simulink model "test3"  (Simulink 7.5)
settings: Solver=ode45  StartTime=0.0  StopTime=10.0  RelTol=1e-3
InitFcn:
  | %% DSPBuilder Start
  | alt_dspbuilder_update_model(bdroot)
  | %% DSPBuilder End
libraries: allblocks_alteradspbuilder2 x16
settings Model: Creator=Administrator  LastModifiedBy=Administrator

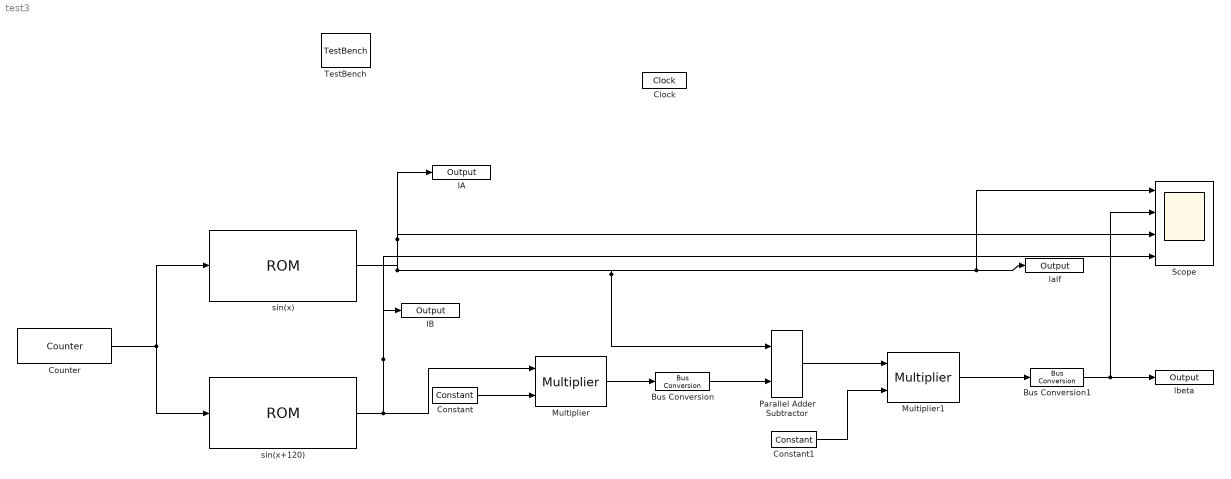
== system test3 ==
  Bus Conversion : allblocks_alteradspbuilder2/Bus Conversion  BusType=Signed Fractional  ibwl=18  ibwr=14  bwl=2  bwr=14  bitToConnectToOutputLSB=3  round=off  saturate=off  pipeline_display=0
  Bus Conversion1 : allblocks_alteradspbuilder2/Bus Conversion  BusType=Signed Fractional  ibwl=4  ibwr=28  bwl=2  bwr=14  bitToConnectToOutputLSB=3  round=off  saturate=off  pipeline_display=0
  Clock : allblocks_alteradspbuilder2/Clock  ClockPeriod=1/10000  ClockPeriodUnit=sec  SampleTime=1/10000  ResetLatency=0  ResetRegisterCascadeDepth=0  SimulationStartCycle=5  PhaseOffset=0  Reset=aclr  ResetType=Active Low  Export=off
  Constant : allblocks_alteradspbuilder2/Constant  mask_cst=2  BusType=Signed Integer  bwl=16  bwr=0  roundMode=Truncate  satMode=Wrap  SpecifyClock=off  allowFloatingPointOverride=on  logOutputs=off  logFile=C:\altera\13.1\quartus\dsp_builder\tb_test3\test3_Constant.fixedpointlog
  Constant1 : allblocks_alteradspbuilder2/Constant  mask_cst=sqrt(1/3)  BusType=Signed Fractional  bwl=2  bwr=14  roundMode=Truncate  satMode=Wrap  SpecifyClock=off  allowFloatingPointOverride=on  logOutputs=off  logFile=C:\altera\13.1\quartus\dsp_builder\tb_test3\test3_Constant1.fixedpointlog
  Counter : allblocks_alteradspbuilder2/Counter  BusType=Unsigned Integer  bwl=12  bwr=0  use_modulo=on  modulo=4096  SpecifyClock=off  direction=Increment  use_sload=off  use_sset=off  svalue=1  use_clk_ena=off  use_ena=off  use_sclr=off  pipeline_display=1
  IA : allblocks_alteradspbuilder2/Output  iofile=C:\altera\13.1\quartus\dsp_builder\tb_test3\test3_IA.capture  BusType=Signed Fractional  bwl=2  bwr=14  externalType=Inferred  PORTTYPE=Output  allowFloatingPointOverride=on  logOutputs=off
  IB : allblocks_alteradspbuilder2/Output  iofile=C:\altera\13.1\quartus\dsp_builder\tb_test3\test3_IB.capture  BusType=Signed Fractional  bwl=2  bwr=14  externalType=Inferred  PORTTYPE=Output  allowFloatingPointOverride=on  logOutputs=off
  Multiplier : allblocks_alteradspbuilder2/Multiplier  BusType=Signed Fractional  bwl=2  bwr=14  pipeline=0  pipeline_display=0  allowFloatingPointOverride=on  logOutputs=off  logFile=C:\altera\13.1\quartus\dsp_builder\tb_test3\test3_Multiplier.fixedpointlog  UseEqualInputWidth=off  bbwl=16  bbwr=0  FullResolution=on  OutputMsb=8  OutputLsb=0  OutputBwl=16  OutputBwr=16  UseDedicatedCircuitry=YES  use_ena=off  use_aclr=off
  Multiplier1 : allblocks_alteradspbuilder2/Multiplier  BusType=Signed Fractional  bwl=2  bwr=14  pipeline=0  pipeline_display=0  allowFloatingPointOverride=on  logOutputs=off  logFile=C:\altera\13.1\quartus\dsp_builder\tb_test3\test3_Multiplier1.fixedpointlog  UseEqualInputWidth=off  bbwl=2  bbwr=14  FullResolution=on  OutputMsb=8  OutputLsb=0  OutputBwl=16  OutputBwr=16  UseDedicatedCircuitry=YES  use_ena=off  use_aclr=off
  Parallel Adder Subtractor : allblocks_alteradspbuilder2/Parallel Adder Subtractor  number_of_inputs=2  direction=++  use_pipeline=on  pipeline_display=1  phase_selection=1  use_ena=off  use_aclr=off  allowFloatingPointOverride=on  logOutputs=off  logFile=C:\altera\13.1\quartus\dsp_builder\tb_test3\test3_Parallel+Adder+Subtractor.fixedpointlog
  Scope : Scope  NumInputPorts=4
      settings: YMin=-1~-1.25~-1~-1  YMax=1~1~1~1
  TestBench : allblocks_alteradspbuilder2/TestBench  enable=on  advancedMode=off  modelSimGui=off  maxDisplayErrors=10  mismatchErrorLevel=Error  simdatafile=C:\altera\13.1\quartus\dsp_builder\tb_test3\test3.simdata.tcl
  lalf : allblocks_alteradspbuilder2/Output  iofile=C:\altera\13.1\quartus\dsp_builder\tb_test3\test3_lalf.capture  BusType=Signed Fractional  bwl=2  bwr=14  externalType=Inferred  PORTTYPE=Output  allowFloatingPointOverride=on  logOutputs=off
  lbeta : allblocks_alteradspbuilder2/Output  iofile=C:\altera\13.1\quartus\dsp_builder\tb_test3\test3_lbeta.capture  BusType=Signed Fractional  bwl=2  bwr=14  externalType=Inferred  PORTTYPE=Output  allowFloatingPointOverride=on  logOutputs=off
  sin(x) : allblocks_alteradspbuilder2/ROM  numwords=4096  BusType=Signed Fractional  bwl=2  bwr=14  memory_type=M9K  ram_type=ROM  initialization=From MATLAB array  init_file=input.hex  init_array=sin([0:2*pi/(2^12):2*pi])  register_outputs=off  use_ena=off  ClockPhase=1  pipeline_display=1  allowFloatingPointOverride=on  logOutputs=off  logFile=C:\altera\13.1\quartus\dsp_builder\tb_test3\test3_sin%28x%29.fixedpointlog  enable_runtime_mod=off  instance_name=AAAA
  sin(x+120) : allblocks_alteradspbuilder2/ROM  numwords=4096  BusType=Signed Fractional  bwl=2  bwr=14  memory_type=M9K  ram_type=ROM  initialization=From MATLAB array  init_file=input.hex  init_array=sin([0:2*pi/(2^12):2*pi]-2*pi/3)  register_outputs=off  use_ena=off  ClockPhase=1  pipeline_display=1  allowFloatingPointOverride=on  logOutputs=off  logFile=C:\altera\13.1\quartus\dsp_builder\tb_test3\test3_sin%28x%2B120%29.fixedpointlog  enable_runtime_mod=off  instance_name=AAAA
  wires:
  Counter/1 -> sin(x)/1, sin(x+120)/1
  sin(x)/1 -> Parallel Adder Subtractor/1, lalf/1, Scope/1, IA/1, Scope/3
  Constant/1 -> Multiplier/2
  Multiplier/1 -> Bus Conversion/1
  Bus Conversion/1 -> Parallel Adder Subtractor/2
  Constant1/1 -> Multiplier1/2
  Parallel Adder Subtractor/1 -> Multiplier1/1
  Multiplier1/1 -> Bus Conversion1/1
  Bus Conversion1/1 -> lbeta/1, Scope/2
  sin(x+120)/1 -> Multiplier/1, IB/1, Scope/4
